simulink model "Din25"  (R2015a)
settings: Solver=ode4  StartTime=0.0  StopTime=10.0  FixedStep=1e-3  RelTol=1e-3
settings Model: Creator=HP  LastModifiedBy=HP

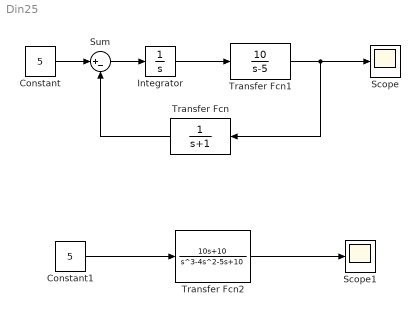
== system Din25 ==
  Constant : Constant  Value=5
  Constant1 : Constant  Value=5
  Integrator : Integrator
  Scope : Scope
      settings: SaveName=dy
  Scope1 : Scope
      settings: SaveName=sd
  Sum : Sum  Inputs=|+-
  Transfer Fcn : TransferFcn  Denominator=[1 1]
  Transfer Fcn1 : TransferFcn  Numerator=[10]  Denominator=[1 -5]
  Transfer Fcn2 : TransferFcn  Numerator=[10 10]  Denominator=[1 -4 -5 10]
  wires:
  Constant/1 -> Sum/1
  Sum/1 -> Integrator/1
  Integrator/1 -> Transfer Fcn1/1
  Transfer Fcn1/1 -> Scope/1, Transfer Fcn/1
  Transfer Fcn/1 -> Sum/2
  Constant1/1 -> Transfer Fcn2/1
  Transfer Fcn2/1 -> Scope1/1
